simulink model "simMA"  (R2018b)
settings: Solver=FixedStepAuto  StartTime=0.0  StopTime=100  FixedStep=0.001  RelTol=1e-3
values from neighbouring files (symbols this model uses):
  A = [-a1/A1 a1/A1;a1/A2 -1*(a1+a2)/A2]    [script8.m]
  B = [1/A1 0;0 1/A2]    [script8.m]
  C = [1 0;0 1]    [script8.m]
  D = [0 0;0 0]    [script8.m]
  dfwe1 = 0.1 * fwe1max    [script8.m]
  dt = 20    [script8.m]
  fwe1 = fwe10(i)    [script8.m]
  fwe2 = 0.2594    [script8.m]
  H0 = [h10; h20]    [script8.m]
settings Model: Creator=wojciechkonury  LastModifiedBy=wojciechkonury

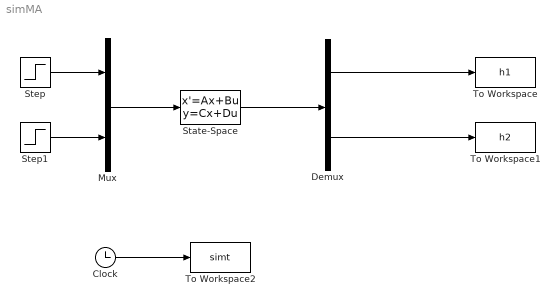
== system simMA ==
  Clock : Clock
  Demux : Demux  Outputs=2
  Mux : Mux  Inputs=2
  State-Space : StateSpace  A=A  B=B  C=C  D=D  InitialCondition=H0
  Step : Step  Time=dt  Before=fwe1  After=fwe1+dfwe1  SampleTime=0
  Step1 : Step  Time=dt  Before=fwe2  After=fwe2  SampleTime=0
  To Workspace : ToWorkspace  VariableName=h1  SampleTime=-1
  To Workspace1 : ToWorkspace  VariableName=h2  SampleTime=-1
  To Workspace2 : ToWorkspace  VariableName=simt  SampleTime=-1
  wires:
  Step1/1 -> Mux/2
  Step/1 -> Mux/1
  Mux/1 -> State-Space/1
  State-Space/1 -> Demux/1
  Demux/1 -> To Workspace/1
  Demux/2 -> To Workspace1/1
  Clock/1 -> To Workspace2/1
